simulink model "joint_space_adaptive"  (R2021b)
settings: Solver=VariableStepAuto  StartTime=0.0  StopTime=10.0  RelTol=1e-3
undefined symbols (not defined in the file): A, F, F_est, G, G_est, I, I_est, KD, Ktheta, lambda
settings Model: Creator=simon  LastModifiedBy=miche
settings SolverCC: AlgebraicLoopSolver=TrustRegion
settings DebuggingCC: SFMachineParentedDataDiag=warning

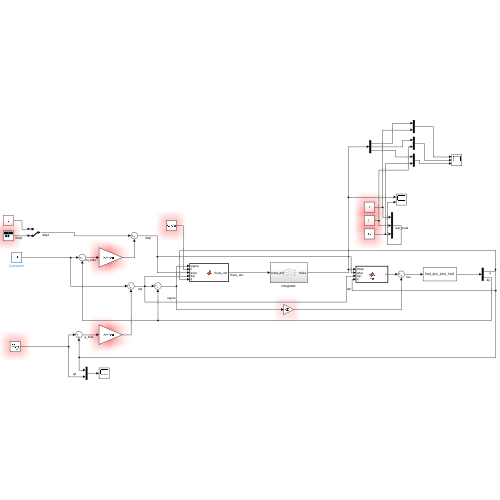
[thumbnail: Simulink's stored preview of the top-level diagram]
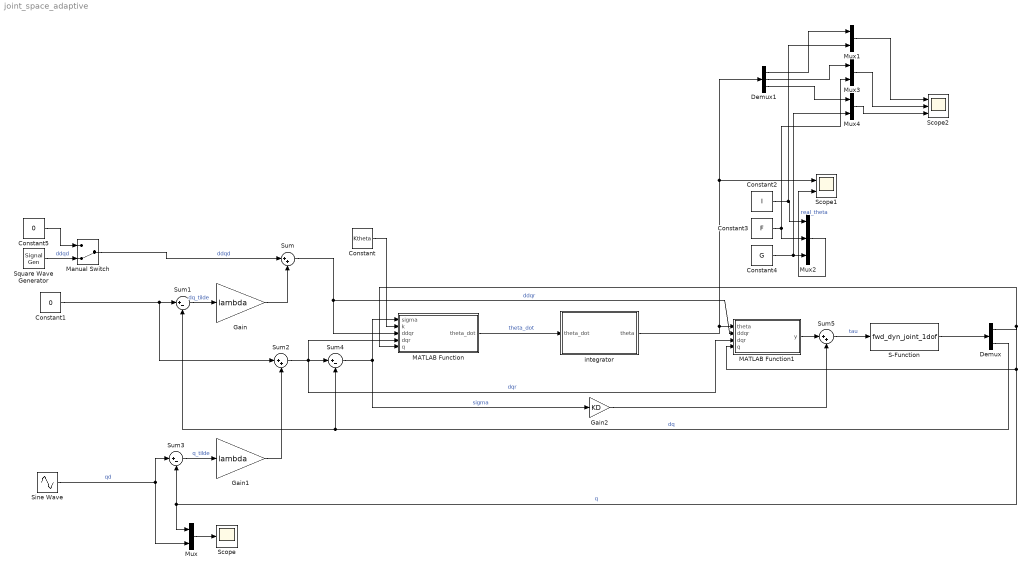
== system joint_space_adaptive ==
  Constant : Constant  Value=Ktheta
  Constant1 : Constant  Value=0
  Constant2 : Constant  Value=I
  Constant3 : Constant  Value=F
  Constant4 : Constant  Value=G
  Constant5 : Constant  Value=0
  Demux : Demux  Outputs=2
  Demux1 : Demux  Outputs=3
  Gain : Gain  Gain=lambda
  Gain1 : Gain  Gain=lambda
  Gain2 : Gain  Gain=KD
  MATLAB Function : MATLAB Function  TreatAsAtomicUnit=on
  MATLAB Function1 : MATLAB Function  TreatAsAtomicUnit=on
  Manual Switch : ManualSwitch  CurrentSetting=0
  Mux{,1,3..4} (4 alike) : Mux  Inputs=2
  Mux2 : Mux  Inputs=3
  S-Function : S-Function  FunctionName=fwd_dyn_joint_1dof  Parameters=qi, dqi,I,F,G  SFunctionDeploymentMode=off  EnableBusSupport=off
  Scope : Scope
  Scope1 : Scope  NumInputPorts=2
  Scope2 : Scope  NumInputPorts=3
  Sine Wave : Sin  Amplitude=A  Frequency=3.14  SampleTime=0
  Square Wave Generator : SignalGenerator  WaveForm=square  Amplitude=A  Units=rad/sec
  Sum : Sum  Inputs=|++
  Sum1 : Sum  Inputs=|+-
  Sum2 : Sum  Inputs=|++
  Sum3 : Sum  Inputs=|+-
  Sum4 : Sum  Inputs=|+-
  Sum5 : Sum  Inputs=|++
  integrator : Subsystem
  wires:
  Manual Switch/1 -> Sum/1  "ddqd"
  Sum1/1 -> Gain/1  "dq_tilde"
  Gain/1 -> Sum/2
  Constant1/1 -> Sum2/1, Sum1/1
  Gain1/1 -> Sum2/2
  Sum3/1 -> Gain1/1  "q_tilde"
  Sine Wave/1 -> Mux/2, Sum3/1  "qd"
  Sum2/1 -> MATLAB Function/4(dqr), Sum4/1, MATLAB Function1/3(dqr)  "dqr"
  Sum4/1 -> MATLAB Function/1(sigma), Gain2/1  "sigma"
  MATLAB Function1/1(y) -> Sum5/1
  S-Function/1 -> Demux/1
  Demux/1 -> Sum3/2, Mux/1, MATLAB Function1/4(q), MATLAB Function/5(q)  "q"
  Demux/2 -> Sum1/2, Sum4/2  "dq"
  Gain2/1 -> Sum5/2
  Sum/1 -> MATLAB Function/3(ddqr), MATLAB Function1/2(ddqr)  "ddqr"
  Constant/1 -> MATLAB Function/2(k)
  Mux/1 -> Scope/1
  Sum5/1 -> S-Function/1  "tau"
  Constant2/1 -> Mux1/2, Mux2/1
  Constant3/1 -> Mux2/2, Mux3/2
  Constant4/1 -> Mux4/2, Mux2/3
  Mux2/1 -> Scope1/2  "real_theta"
  integrator/1(theta) -> Demux1/1, Scope1/1, MATLAB Function1/1(theta)
  MATLAB Function/1(theta_dot) -> integrator/1(theta_dot)  "theta_dot"
  Constant5/1 -> Manual Switch/1
  Square Wave Generator/1 -> Manual Switch/2  "ddqd"
  Demux1/1 -> Mux1/1
  Demux1/2 -> Mux3/1
  Demux1/3 -> Mux4/1
  Mux1/1 -> Scope2/1
  Mux3/1 -> Scope2/2
  Mux4/1 -> Scope2/3

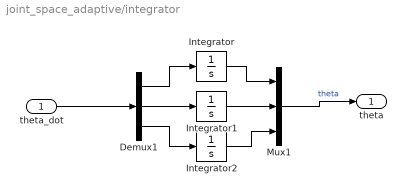
== system joint_space_adaptive/integrator ==
  theta_dot : Inport
  Demux1 : Demux  Outputs=3
  Integrator : Integrator  InitialCondition=I_est
  Integrator1 : Integrator  InitialCondition=F_est
  Integrator2 : Integrator  InitialCondition=G_est
  Mux1 : Mux  Inputs=3
  theta : Outport
  wires:
  Integrator/1 -> Mux1/1
  Integrator1/1 -> Mux1/2
  theta_dot/1 -> Demux1/1
  Integrator2/1 -> Mux1/3
  Demux1/2 -> Integrator1/1
  Demux1/3 -> Integrator2/1
  Demux1/1 -> Integrator/1
  Mux1/1 -> theta/1  "theta"

== matlab function joint_space_adaptive/MATLAB Function1 ==
  data: theta input; y output; ddqr input; dqr input; q input
function y = fcn(theta, ddqr, dqr, q)

y = [ddqr dqr sin(q)]*theta;

== matlab function joint_space_adaptive/MATLAB Function ==
  data: sigma input; k input; theta_dot output size=3; ddqr input; dqr input; q input
function theta_dot = fcn(sigma,k,ddqr,dqr,q)

theta_dot = k*[ddqr;dqr;sin(q)];
